simulink model "CM"  (R2017b)
settings: Solver=VariableStepAuto  StartTime=0.0  StopTime=10.0  RelTol=1e-3
values from neighbouring files (symbols this model uses):
  CMadot = -7.27    [Cessna_Simulation.m]
  CMel = -1.122    [Cessna_Simulation.m]
  CMq = -12.4    [Cessna_Simulation.m]
undefined symbols (not defined in the file or in its folder): cbar, CM0, CMa
settings Model: Creator=stroll  LastModifiedBy=stroll

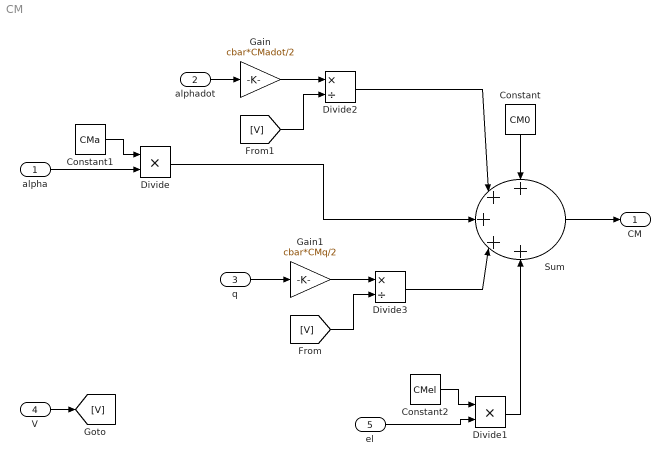
== system CM ==
  alpha : Inport
  alphadot : Inport  Port=2
  q : Inport  Port=3
  V : Inport  Port=4
  el : Inport  Port=5
  Constant : Constant  Value=CM0
  Constant1 : Constant  Value=CMa
  Constant2 : Constant  Value=CMel
  Divide : Product
  Divide1 : Product
  Divide2 : Product  Inputs=*/
  Divide3 : Product  Inputs=*/
  Gain : Gain  Gain=cbar*CMadot/2
  Gain1 : Gain  Gain=cbar*CMq/2
  Sum : Sum  Inputs=+++++
  CM : Outport
  wires:
  Constant/1 -> Sum/1
  [V] -> Divide3/2
  Divide2/1 -> Sum/2
  Gain1/1 -> Divide3/1
  Divide/1 -> Sum/3
  Constant2/1 -> Divide1/1
  el/1 -> Divide1/2
  V/1 -> [V]
  [V] -> Divide2/2
  Sum/1 -> CM/1
  Constant1/1 -> Divide/1
  Divide1/1 -> Sum/5
  q/1 -> Gain1/1
  Gain/1 -> Divide2/1
  alphadot/1 -> Gain/1
  alpha/1 -> Divide/2
  Divide3/1 -> Sum/4
